simulink model "VTOL_RESPONSE_SIMULINK_MEX"  (R2024b)
settings: Solver=FixedStepDiscrete  StartTime=0.0  StopTime=2.0  FixedStep=dt_sim  RelTol=1e-3
InitFcn:
  | SETUP_FAST_DISK_MEX_BASE;
values from neighbouring files (symbols this model uses):
  rotor_state0 = zeros(n_rotors * response_rotor_state_size, 1)    [RUN_RESPONSE_SIMULINK_SETUP.m]
  rotor_tilt_angle_deg = trim_rotor_tilt_angle_deg(:)    [RUN_RESPONSE_SIMULINK_SETUP.m]
  x0 = trim_results.response.state_history(1,:).'    [RUN_RESPONSE_SIMULINK_SETUP.m]
undefined symbols (not defined in the file or in its folder): control_delta, dt_sim, fixed_control_delta, pilot_stick, pilot_stick_to_control_gain_deg
settings Model: Creator=yuany  LastModifiedBy=yuany

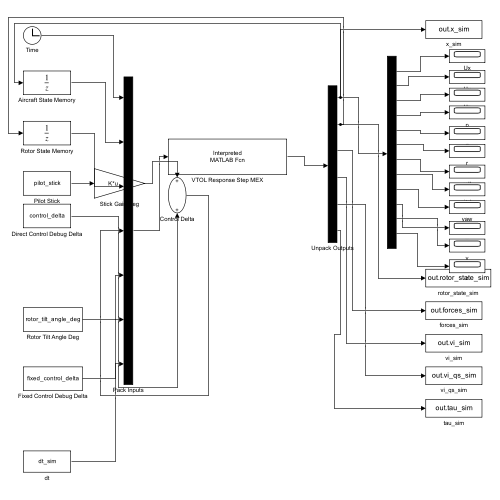
[thumbnail: Simulink's stored preview of the top-level diagram]
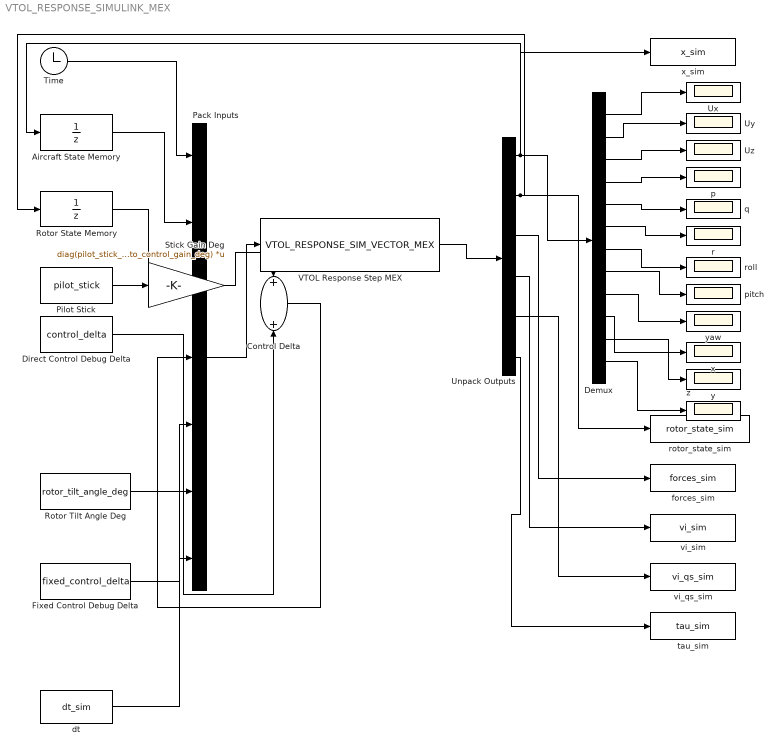
== system VTOL_RESPONSE_SIMULINK_MEX ==
  Aircraft State Memory : UnitDelay  InitialCondition=x0  SampleTime=dt_sim  HasFrameUpgradeWarning=on
  Control Delta : Sum
  Demux : Demux  Outputs=12
  Direct Control Debug Delta : Constant  Value=control_delta  SampleTime=dt_sim
  Fixed Control Debug Delta : Constant  Value=fixed_control_delta  SampleTime=dt_sim
  Pack Inputs : Mux  Inputs=7
  Pilot Stick : Constant  Value=pilot_stick  SampleTime=dt_sim
  Rotor State Memory : UnitDelay  InitialCondition=rotor_state0  SampleTime=dt_sim  HasFrameUpgradeWarning=on
  Rotor Tilt Angle Deg : Constant  Value=rotor_tilt_angle_deg  SampleTime=dt_sim
  Stick Gain Deg : Gain  Gain=diag(pilot_stick_to_control_gain_deg)  Multiplication=Matrix(K*u)
  Time : Clock
  Unpack Outputs : Demux  Outputs=[12 42 6 6 6 6]
  Ux : Scope
  Uy : Scope
  Uz : Scope
  VTOL Response Step MEX : MATLABFcn  MATLABFcn=VTOL_RESPONSE_SIM_VECTOR_MEX  OutputDimensions=78  SampleTime=dt_sim
  dt : Constant  Value=dt_sim  SampleTime=dt_sim
  forces_sim : ToWorkspace  VariableName=forces_sim  SaveFormat=Structure With Time  SampleTime=-1
  p : Scope
  pitch : Scope
  q : Scope
  r : Scope
  roll : Scope
  rotor_state_sim : ToWorkspace  VariableName=rotor_state_sim  SaveFormat=Structure With Time  SampleTime=-1
  tau_sim : ToWorkspace  VariableName=tau_sim  SaveFormat=Structure With Time  SampleTime=-1
  vi_qs_sim : ToWorkspace  VariableName=vi_qs_sim  SaveFormat=Structure With Time  SampleTime=-1
  vi_sim : ToWorkspace  VariableName=vi_sim  SaveFormat=Structure With Time  SampleTime=-1
  x : Scope
  x_sim : ToWorkspace  VariableName=x_sim  SaveFormat=Structure With Time  SampleTime=-1
  y : Scope
  yaw : Scope
  z : Scope
  wires:
  Time/1 -> Pack Inputs/1
  Aircraft State Memory/1 -> Pack Inputs/2
  Rotor State Memory/1 -> Pack Inputs/3
  Pilot Stick/1 -> Stick Gain Deg/1
  Stick Gain Deg/1 -> Control Delta/1
  Direct Control Debug Delta/1 -> Control Delta/2
  Control Delta/1 -> Pack Inputs/4
  Rotor Tilt Angle Deg/1 -> Pack Inputs/5
  Fixed Control Debug Delta/1 -> Pack Inputs/6
  dt/1 -> Pack Inputs/7
  Pack Inputs/1 -> VTOL Response Step MEX/1
  VTOL Response Step MEX/1 -> Unpack Outputs/1
  Unpack Outputs/1 -> Aircraft State Memory/1, x_sim/1, Demux/1
  Unpack Outputs/2 -> Rotor State Memory/1, rotor_state_sim/1
  Unpack Outputs/3 -> forces_sim/1
  Unpack Outputs/4 -> vi_sim/1
  Unpack Outputs/5 -> vi_qs_sim/1
  Unpack Outputs/6 -> tau_sim/1
  Demux/1 -> Ux/1
  Demux/2 -> Uy/1
  Demux/3 -> Uz/1
  Demux/4 -> p/1
  Demux/5 -> q/1
  Demux/6 -> r/1
  Demux/7 -> roll/1
  Demux/8 -> pitch/1
  Demux/9 -> yaw/1
  Demux/10 -> x/1
  Demux/11 -> y/1
  Demux/12 -> z/1
